simulink model "PassengerCar"  (R2019b)
settings: Solver=ode1  StartTime=0  StopTime=25  FixedStep=1.0000000000000000e-003  RelTol=1e-3
InitFcn:
  | sampleTime = str2double(get_param(bdroot, 'FixedStep'));
undefined symbols (not defined in the file or in its folder): AccPedalPos, BrakePedalPos, BrakeSwitch, DiscIntNeverNeededParam, DYNA4, EngSpd, IgnitionSwitch, InitialGear, InitialSpeed, IntendedEngTrq, LeftIndicator, MainBrakePress, MaxGear, MDL, MinGear, RefAcc, RefLane, RefLatPos, RefPath, RefPathCurv, RefSpd, RefSpdPreview, RefSpdRetrospect, RightIndicator, SteeringWheelAng, SteeringWheelTrq, UserDefinedRefValue, vm_const
libraries: UtilitiesLibrary x31, simulink x18, WheelSystemModules x13, LongitudinalControllerModules x13, LateralControllerModules x7, AnimationBusselectorModules x5, EnvironmentModules x5, BasicEngineControlModules x5, MiscellaneousControlModules x5, Animation3Modules x4, AuxiliariesModules x4, TireModules x4
(part 32 of 39)

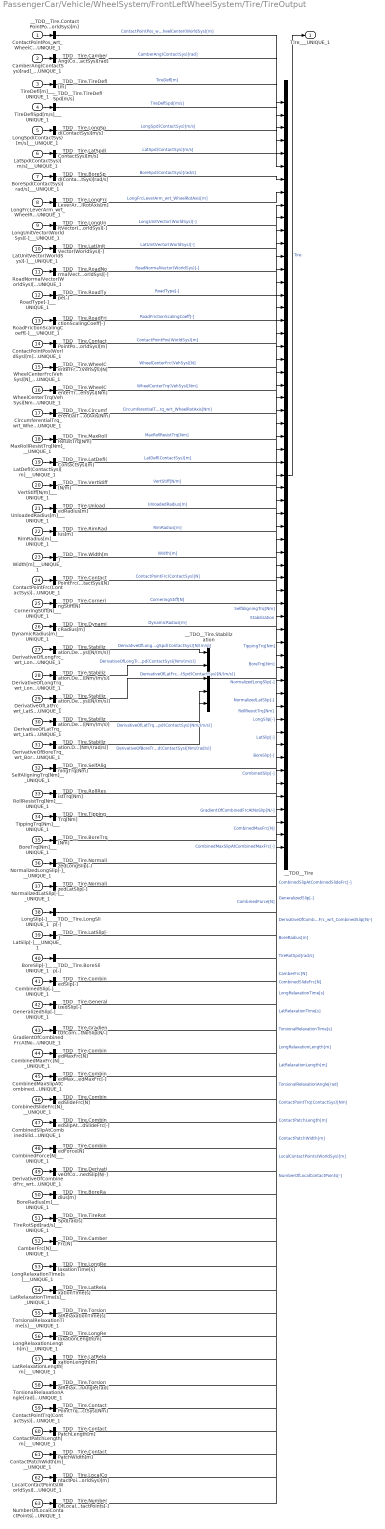
== system PassengerCar/Vehicle/WheelSystem/FrontLeftWheelSystem/Tire/TireOutput ==
  ContactPointPos_wrt_WheelCenter(WorldSys)[m]___UNIQUE_1 : Inport  Description=|  PortDimensions=[3]
      | <name>ContactPointPos_wrt_WheelCenter(WorldSys)[m]</name>
      | <comment></comment>
  CamberAng(ContactSys)[rad]___UNIQUE_1 : Inport  Description=|  Port=2  PortDimensions=[1]
      | <name>CamberAng(ContactSys)[rad]</name>
      | <comment></comment>
  TireDefl[m]___UNIQUE_1 : Inport  Description=|  Port=3  PortDimensions=[1]
      | <name>TireDefl[m]</name>
      | <comment></comment>
  TireDeflSpd[m/s]___UNIQUE_1 : Inport  Description=|  Port=4  PortDimensions=[1]
      | <name>TireDeflSpd[m/s]</name>
      | <comment></comment>
  LongSpd(ContactSys)[m/s]___UNIQUE_1 : Inport  Description=|  Port=5  PortDimensions=[1]
      | <name>LongSpd(ContactSys)[m/s]</name>
      | <comment></comment>
  LatSpd(ContactSys)[m/s]___UNIQUE_1 : Inport  Description=|  Port=6  PortDimensions=[1]
      | <name>LatSpd(ContactSys)[m/s]</name>
      | <comment></comment>
  BoreSpd(ContactSys)[rad/s]___UNIQUE_1 : Inport  Description=|  Port=7  PortDimensions=[1]
      | <name>BoreSpd(ContactSys)[rad/s]</name>
      | <comment></comment>
  LongFrcLeverArm_wrt_WheelRotAxis[m]___UNIQUE_1 : Inport  Description=|  Port=8  PortDimensions=[1]
      | <name>LongFrcLeverArm_wrt_WheelRotAxis[m]</name>
      | <comment></comment>
  LongUnitVector(WorldSys)[-]___UNIQUE_1 : Inport  Description=|  Port=9  PortDimensions=[3]
      | <name>LongUnitVector(WorldSys)[-]</name>
      | <comment></comment>
  LatUnitVector(WorldSys)[-]___UNIQUE_1 : Inport  Description=|  Port=10  PortDimensions=[3]
      | <name>LatUnitVector(WorldSys)[-]</name>
      | <comment></comment>
  RoadNormalVector(WorldSys)[-]___UNIQUE_1 : Inport  Description=|  Port=11  PortDimensions=[3]
      | <name>RoadNormalVector(WorldSys)[-]</name>
      | <comment></comment>
  RoadType[-]___UNIQUE_1 : Inport  Description=|  Port=12  PortDimensions=[1]
      | <name>RoadType[-]</name>
      | <comment></comment>
  RoadFrictionScalingCoeff[-]___UNIQUE_1 : Inport  Description=|  Port=13  PortDimensions=[1]
      | <name>RoadFrictionScalingCoeff[-]</name>
      | <comment></comment>
  ContactPointPos(WorldSys)[m]___UNIQUE_1 : Inport  Description=|  Port=14  PortDimensions=[3]
      | <name>ContactPointPos(WorldSys)[m]</name>
      | <comment></comment>
  WheelCenterFrc(VehSys)[N]___UNIQUE_1 : Inport  Description=|  Port=15  PortDimensions=[3]
      | <name>WheelCenterFrc(VehSys)[N]</name>
      | <comment></comment>
  WheelCenterTrq(VehSys)[Nm]___UNIQUE_1 : Inport  Description=|  Port=16  PortDimensions=[3]
      | <name>WheelCenterTrq(VehSys)[Nm]</name>
      | <comment></comment>
  CircumferentialTrq_wrt_WheelRotAxis[Nm]___UNIQUE_1 : Inport  Description=|  Port=17  PortDimensions=[1]
      | <name>CircumferentialTrq_wrt_WheelRotAxis[Nm]</name>
      | <comment></comment>
  MaxRollResistTrq[Nm]___UNIQUE_1 : Inport  Description=|  Port=18  PortDimensions=[1]
      | <name>MaxRollResistTrq[Nm]</name>
      | <comment></comment>
  LatDefl(ContactSys)[m]___UNIQUE_1 : Inport  Description=|  Port=19  PortDimensions=[1]
      | <name>LatDefl(ContactSys)[m]</name>
      | <comment></comment>
  VertStiff[N/m]___UNIQUE_1 : Inport  Description=|  Port=20  PortDimensions=[1]
      | <name>VertStiff[N/m]</name>
      | <comment></comment>
  UnloadedRadius[m]___UNIQUE_1 : Inport  Description=|  Port=21  PortDimensions=[1]
      | <name>UnloadedRadius[m]</name>
      | <comment></comment>
  RimRadius[m]___UNIQUE_1 : Inport  Description=|  Port=22  PortDimensions=[1]
      | <name>RimRadius[m]</name>
      | <comment></comment>
  Width[m]___UNIQUE_1 : Inport  Description=|  Port=23  PortDimensions=[1]
      | <name>Width[m]</name>
      | <comment></comment>
  ContactPointFrc(ContactSys)[N]___UNIQUE_1 : Inport  Description=|  Port=24  PortDimensions=[3]
      | <name>ContactPointFrc(ContactSys)[N]</name>
      | <comment></comment>
  CorneringStiff[N]___UNIQUE_1 : Inport  Description=|  Port=25  PortDimensions=[1]
      | <name>CorneringStiff[N]</name>
      | <comment></comment>
  DynamicRadius[m]___UNIQUE_1 : Inport  Description=|  Port=26  PortDimensions=[1]
      | <name>DynamicRadius[m]</name>
      | <comment></comment>
  DerivativeOfLongFrc_wrt_LongSpd(ContactSys)[N/(m/s)]___UNIQUE_1 : Inport  Description=|  Port=27  PortDimensions=[1]
      | <name>Stabilization.DerivativeOfLongFrc_wrt_LongSpd(ContactSys)[N/(m/s)]</name>
      | <comment></comment>
  DerivativeOfLongTrq_wrt_LongSpd(ContactSys)[Nm/(m/s)]___UNIQUE_1 : Inport  Description=|  Port=28  PortDimensions=[1]
      | <name>Stabilization.DerivativeOfLongTrq_wrt_LongSpd(ContactSys)[Nm/(m/s)]</name>
      | <comment></comment>
  DerivativeOfLatFrc_wrt_LatSpd(ContactSys)[N/(m/s)]___UNIQUE_1 : Inport  Description=|  Port=29  PortDimensions=[1]
      | <name>Stabilization.DerivativeOfLatFrc_wrt_LatSpd(ContactSys)[N/(m/s)]</name>
      | <comment></comment>
  DerivativeOfLatTrq_wrt_LatSpd(ContactSys)[Nm/(m/s)]___UNIQUE_1 : Inport  Description=|  Port=30  PortDimensions=[1]
      | <name>Stabilization.DerivativeOfLatTrq_wrt_LatSpd(ContactSys)[Nm/(m/s)]</name>
      | <comment></comment>
  DerivativeOfBoreTrq_wrt_BoreSpd(ContactSys)[Nm/(rad/s)]___UNIQUE_1 : Inport  Description=|  Port=31  PortDimensions=[1]
      | <name>Stabilization.DerivativeOfBoreTrq_wrt_BoreSpd(ContactSys)[Nm/(rad/s)]</name>
      | <comment></comment>
  SelfAligningTrq[Nm]___UNIQUE_1 : Inport  Description=|  Port=32  PortDimensions=[1]
      | <name>SelfAligningTrq[Nm]</name>
      | <comment></comment>
  RollResistTrq[Nm]___UNIQUE_1 : Inport  Description=|  Port=33  PortDimensions=[1]
      | <name>RollResistTrq[Nm]</name>
      | <comment></comment>
  TippingTrq[Nm]___UNIQUE_1 : Inport  Description=|  Port=34  PortDimensions=[1]
      | <name>TippingTrq[Nm]</name>
      | <comment></comment>
  BoreTrq[Nm]___UNIQUE_1 : Inport  Description=|  Port=35  PortDimensions=[1]
      | <name>BoreTrq[Nm]</name>
      | <comment></comment>
  NormalizedLongSlip[-]___UNIQUE_1 : Inport  Description=|  Port=36  PortDimensions=[1]
      | <name>NormalizedLongSlip[-]</name>
      | <comment></comment>
  NormalizedLatSlip[-]___UNIQUE_1 : Inport  Description=|  Port=37  PortDimensions=[1]
      | <name>NormalizedLatSlip[-]</name>
      | <comment></comment>
  LongSlip[-]___UNIQUE_1 : Inport  Description=|  Port=38  PortDimensions=[1]
      | <name>LongSlip[-]</name>
      | <comment></comment>
  LatSlip[-]___UNIQUE_1 : Inport  Description=|  Port=39  PortDimensions=[1]
      | <name>LatSlip[-]</name>
      | <comment></comment>
  BoreSlip[-]___UNIQUE_1 : Inport  Description=|  Port=40  PortDimensions=[1]
      | <name>BoreSlip[-]</name>
      | <comment></comment>
  CombinedSlip[-]___UNIQUE_1 : Inport  Description=|  Port=41  PortDimensions=[1]
      | <name>CombinedSlip[-]</name>
      | <comment></comment>
  GeneralizedSlip[-]___UNIQUE_1 : Inport  Description=|  Port=42  PortDimensions=[1]
      | <name>GeneralizedSlip[-]</name>
      | <comment></comment>
  GradientOfCombinedFrcAtNoSlip[N/-]___UNIQUE_1 : Inport  Description=|  Port=43  PortDimensions=[1]
      | <name>GradientOfCombinedFrcAtNoSlip[N/-]</name>
      | <comment></comment>
  CombinedMaxFrc[N]___UNIQUE_1 : Inport  Description=|  Port=44  PortDimensions=[1]
      | <name>CombinedMaxFrc[N]</name>
      | <comment></comment>
  CombinedMaxSlipAtCombinedMaxFrc[-]___UNIQUE_1 : Inport  Description=|  Port=45  PortDimensions=[1]
      | <name>CombinedMaxSlipAtCombinedMaxFrc[-]</name>
      | <comment></comment>
  CombinedSlideFrc[N]___UNIQUE_1 : Inport  Description=|  Port=46  PortDimensions=[1]
      | <name>CombinedSlideFrc[N]</name>
      | <comment></comment>
  CombinedSlipAtCombinedSlideFrc[-]___UNIQUE_1 : Inport  Description=|  Port=47  PortDimensions=[1]
      | <name>CombinedSlipAtCombinedSlideFrc[-]</name>
      | <comment></comment>
  CombinedForce[N]___UNIQUE_1 : Inport  Description=|  Port=48  PortDimensions=[1]
      | <name>CombinedForce[N]</name>
      | <comment></comment>
  DerivativeOfCombinedFrc_wrt_CombinedSlip[N/-]___UNIQUE_1 : Inport  Description=|  Port=49  PortDimensions=[1]
      | <name>DerivativeOfCombinedFrc_wrt_CombinedSlip[N/-]</name>
      | <comment></comment>
  BoreRadius[m]___UNIQUE_1 : Inport  Description=|  Port=50  PortDimensions=[1]
      | <name>BoreRadius[m]</name>
      | <comment></comment>
  TireRotSpd[rad/s]___UNIQUE_1 : Inport  Description=|  Port=51  PortDimensions=[1]
      | <name>TireRotSpd[rad/s]</name>
      | <comment></comment>
  CamberFrc[N]___UNIQUE_1 : Inport  Description=|  Port=52  PortDimensions=[1]
      | <name>CamberFrc[N]</name>
      | <comment></comment>
  LongRelaxationTime[s]___UNIQUE_1 : Inport  Description=|  Port=53  PortDimensions=[1]
      | <name>LongRelaxationTime[s]</name>
      | <comment></comment>
  LatRelaxationTime[s]___UNIQUE_1 : Inport  Description=|  Port=54  PortDimensions=[1]
      | <name>LatRelaxationTime[s]</name>
      | <comment></comment>
  TorsionalRelaxationTime[s]___UNIQUE_1 : Inport  Description=|  Port=55  PortDimensions=[1]
      | <name>TorsionalRelaxationTime[s]</name>
      | <comment></comment>
  LongRelaxationLength[m]___UNIQUE_1 : Inport  Description=|  Port=56  PortDimensions=[1]
      | <name>LongRelaxationLength[m]</name>
      | <comment></comment>
  LatRelaxationLength[m]___UNIQUE_1 : Inport  Description=|  Port=57  PortDimensions=[1]
      | <name>LatRelaxationLength[m]</name>
      | <comment></comment>
  TorsionalRelaxationAngle[rad]___UNIQUE_1 : Inport  Description=|  Port=58  PortDimensions=[1]
      | <name>TorsionalRelaxationAngle[rad]</name>
      | <comment></comment>
  ContactPointTrq(ContactSys)[Nm]___UNIQUE_1 : Inport  Description=|  Port=59  PortDimensions=[3]
      | <name>ContactPointTrq(ContactSys)[Nm]</name>
      | <comment></comment>
  ContactPatchLength[m]___UNIQUE_1 : Inport  Description=|  Port=60  PortDimensions=[1]
      | <name>ContactPatchLength[m]</name>
      | <comment></comment>
  ContactPatchWidth[m]___UNIQUE_1 : Inport  Description=|  Port=61  PortDimensions=[1]
      | <name>ContactPatchWidth[m]</name>
      | <comment></comment>
  LocalContactPoints(WorldSys)[m]___UNIQUE_1 : Inport  Description=|  Port=62  PortDimensions=[12]
      | <name>LocalContactPoints(WorldSys)[m]</name>
      | <comment></comment>
  NumberOfLocalContactPoints[-]___UNIQUE_1 : Inport  Description=|  Port=63  PortDimensions=[1]
      | <name>NumberOfLocalContactPoints[-]</name>
      | <comment></comment>
  __TDD__Tire.BoreRadius[m] : Demux  Outputs=[1]
  __TDD__Tire.BoreSlip[-] : Demux  Outputs=[1]
  __TDD__Tire.BoreSpd(ContactSys)[rad/s] : Demux  Outputs=[1]
  __TDD__Tire.BoreTrq[Nm] : Demux  Outputs=[1]
  __TDD__Tire.CamberAng(ContactSys)[rad] : Demux  Outputs=[1]
  __TDD__Tire.CamberFrc[N] : Demux  Outputs=[1]
  __TDD__Tire.CircumferentialTrq_wrt_WheelRotAxis[Nm] : Demux  Outputs=[1]
  __TDD__Tire.CombinedForce[N] : Demux  Outputs=[1]
  __TDD__Tire.CombinedMaxFrc[N] : Demux  Outputs=[1]
  __TDD__Tire.CombinedMaxSlipAtCombinedMaxFrc[-] : Demux  Outputs=[1]
  __TDD__Tire.CombinedSlideFrc[N] : Demux  Outputs=[1]
  __TDD__Tire.CombinedSlipAtCombinedSlideFrc[-] : Demux  Outputs=[1]
  __TDD__Tire.CombinedSlip[-] : Demux  Outputs=[1]
  __TDD__Tire.ContactPatchLength[m] : Demux  Outputs=[1]
  __TDD__Tire.ContactPatchWidth[m] : Demux  Outputs=[1]
  __TDD__Tire.ContactPointFrc(ContactSys)[N] : Demux  Outputs=[3]
  __TDD__Tire.ContactPointPos(WorldSys)[m] : Demux  Outputs=[3]
  __TDD__Tire.ContactPointPos_wrt_WheelCenter(WorldSys)[m] : Demux  Outputs=[3]
  __TDD__Tire.ContactPointTrq(ContactSys)[Nm] : Demux  Outputs=[3]
  __TDD__Tire.CorneringStiff[N] : Demux  Outputs=[1]
  __TDD__Tire.DerivativeOfCombinedFrc_wrt_CombinedSlip[N/-] : Demux  Outputs=[1]
  __TDD__Tire.DynamicRadius[m] : Demux  Outputs=[1]
  __TDD__Tire.GeneralizedSlip[-] : Demux  Outputs=[1]
  __TDD__Tire.GradientOfCombinedFrcAtNoSlip[N/-] : Demux  Outputs=[1]
  __TDD__Tire.LatDefl(ContactSys)[m] : Demux  Outputs=[1]
  __TDD__Tire.LatRelaxationLength[m] : Demux  Outputs=[1]
  __TDD__Tire.LatRelaxationTime[s] : Demux  Outputs=[1]
  __TDD__Tire.LatSlip[-] : Demux  Outputs=[1]
  __TDD__Tire.LatSpd(ContactSys)[m/s] : Demux  Outputs=[1]
  __TDD__Tire.LatUnitVector(WorldSys)[-] : Demux  Outputs=[3]
  __TDD__Tire.LocalContactPoints(WorldSys)[m] : Demux  Outputs=[12]
  __TDD__Tire.LongFrcLeverArm_wrt_WheelRotAxis[m] : Demux  Outputs=[1]
  __TDD__Tire.LongRelaxationLength[m] : Demux  Outputs=[1]
  __TDD__Tire.LongRelaxationTime[s] : Demux  Outputs=[1]
  __TDD__Tire.LongSlip[-] : Demux  Outputs=[1]
  __TDD__Tire.LongSpd(ContactSys)[m/s] : Demux  Outputs=[1]
  __TDD__Tire.LongUnitVector(WorldSys)[-] : Demux  Outputs=[3]
  __TDD__Tire.MaxRollResistTrq[Nm] : Demux  Outputs=[1]
  __TDD__Tire.NormalizedLatSlip[-] : Demux  Outputs=[1]
  __TDD__Tire.NormalizedLongSlip[-] : Demux  Outputs=[1]
  __TDD__Tire.NumberOfLocalContactPoints[-] : Demux  Outputs=[1]
  __TDD__Tire.RimRadius[m] : Demux  Outputs=[1]
  __TDD__Tire.RoadFrictionScalingCoeff[-] : Demux  Outputs=[1]
  __TDD__Tire.RoadNormalVector(WorldSys)[-] : Demux  Outputs=[3]
  __TDD__Tire.RoadType[-] : Demux  Outputs=[1]
  __TDD__Tire.RollResistTrq[Nm] : Demux  Outputs=[1]
  __TDD__Tire.SelfAligningTrq[Nm] : Demux  Outputs=[1]
  __TDD__Tire.Stabilization.DerivativeOfBoreTrq_wrt_BoreSpd(ContactSys)[Nm/(rad/s)] : Demux  Outputs=[1]
  __TDD__Tire.Stabilization.DerivativeOfLatFrc_wrt_LatSpd(ContactSys)[N/(m/s)] : Demux  Outputs=[1]
  __TDD__Tire.Stabilization.DerivativeOfLatTrq_wrt_LatSpd(ContactSys)[Nm/(m/s)] : Demux  Outputs=[1]
  __TDD__Tire.Stabilization.DerivativeOfLongFrc_wrt_LongSpd(ContactSys)[N/(m/s)] : Demux  Outputs=[1]
  __TDD__Tire.Stabilization.DerivativeOfLongTrq_wrt_LongSpd(ContactSys)[Nm/(m/s)] : Demux  Outputs=[1]
  __TDD__Tire.TippingTrq[Nm] : Demux  Outputs=[1]
  __TDD__Tire.TireDeflSpd[m/s] : Demux  Outputs=[1]
  __TDD__Tire.TireDefl[m] : Demux  Outputs=[1]
  __TDD__Tire.TireRotSpd[rad/s] : Demux  Outputs=[1]
  __TDD__Tire.TorsionalRelaxationAngle[rad] : Demux  Outputs=[1]
  __TDD__Tire.TorsionalRelaxationTime[s] : Demux  Outputs=[1]
  __TDD__Tire.UnloadedRadius[m] : Demux  Outputs=[1]
  __TDD__Tire.VertStiff[N/m] : Demux  Outputs=[1]
  __TDD__Tire.WheelCenterFrc(VehSys)[N] : Demux  Outputs=[3]
  __TDD__Tire.WheelCenterTrq(VehSys)[Nm] : Demux  Outputs=[3]
  __TDD__Tire.Width[m] : Demux  Outputs=[1]
  __TDO__Tire : BusCreator  Inputs=59
  __TDO__Tire.Stabilization : BusCreator  Inputs=5
  Tire___UNIQUE_1 : Outport  Description=|  PortDimensions=[92]  VectorParamsAs1DForOutWhenUnconnected=off
      | <name>ContactPointPos_wrt_WheelCenter(WorldSys)[m]</name>
      | <comment></comment>
  wires:
  ContactPointPos_wrt_WheelCenter(WorldSys)[m]___UNIQUE_1/1 -> __TDD__Tire.ContactPointPos_wrt_WheelCenter(WorldSys)[m]/1
  __TDD__Tire.ContactPointPos_wrt_WheelCenter(WorldSys)[m]/1 -> __TDO__Tire/1  "ContactPointPos_wrt_WheelCenter(WorldSys)[m]"
  CamberAng(ContactSys)[rad]___UNIQUE_1/1 -> __TDD__Tire.CamberAng(ContactSys)[rad]/1
  __TDD__Tire.CamberAng(ContactSys)[rad]/1 -> __TDO__Tire/2  "CamberAng(ContactSys)[rad]"
  TireDefl[m]___UNIQUE_1/1 -> __TDD__Tire.TireDefl[m]/1
  __TDD__Tire.TireDefl[m]/1 -> __TDO__Tire/3  "TireDefl[m]"
  TireDeflSpd[m/s]___UNIQUE_1/1 -> __TDD__Tire.TireDeflSpd[m/s]/1
  __TDD__Tire.TireDeflSpd[m/s]/1 -> __TDO__Tire/4  "TireDeflSpd[m/s]"
  LongSpd(ContactSys)[m/s]___UNIQUE_1/1 -> __TDD__Tire.LongSpd(ContactSys)[m/s]/1
  __TDD__Tire.LongSpd(ContactSys)[m/s]/1 -> __TDO__Tire/5  "LongSpd(ContactSys)[m/s]"
  LatSpd(ContactSys)[m/s]___UNIQUE_1/1 -> __TDD__Tire.LatSpd(ContactSys)[m/s]/1
  __TDD__Tire.LatSpd(ContactSys)[m/s]/1 -> __TDO__Tire/6  "LatSpd(ContactSys)[m/s]"
  BoreSpd(ContactSys)[rad/s]___UNIQUE_1/1 -> __TDD__Tire.BoreSpd(ContactSys)[rad/s]/1
  __TDD__Tire.BoreSpd(ContactSys)[rad/s]/1 -> __TDO__Tire/7  "BoreSpd(ContactSys)[rad/s]"
  LongFrcLeverArm_wrt_WheelRotAxis[m]___UNIQUE_1/1 -> __TDD__Tire.LongFrcLeverArm_wrt_WheelRotAxis[m]/1
  __TDD__Tire.LongFrcLeverArm_wrt_WheelRotAxis[m]/1 -> __TDO__Tire/8  "LongFrcLeverArm_wrt_WheelRotAxis[m]"
  LongUnitVector(WorldSys)[-]___UNIQUE_1/1 -> __TDD__Tire.LongUnitVector(WorldSys)[-]/1
  __TDD__Tire.LongUnitVector(WorldSys)[-]/1 -> __TDO__Tire/9  "LongUnitVector(WorldSys)[-]"
  LatUnitVector(WorldSys)[-]___UNIQUE_1/1 -> __TDD__Tire.LatUnitVector(WorldSys)[-]/1
  __TDD__Tire.LatUnitVector(WorldSys)[-]/1 -> __TDO__Tire/10  "LatUnitVector(WorldSys)[-]"
  RoadNormalVector(WorldSys)[-]___UNIQUE_1/1 -> __TDD__Tire.RoadNormalVector(WorldSys)[-]/1
  __TDD__Tire.RoadNormalVector(WorldSys)[-]/1 -> __TDO__Tire/11  "RoadNormalVector(WorldSys)[-]"
  RoadType[-]___UNIQUE_1/1 -> __TDD__Tire.RoadType[-]/1
  __TDD__Tire.RoadType[-]/1 -> __TDO__Tire/12  "RoadType[-]"
  RoadFrictionScalingCoeff[-]___UNIQUE_1/1 -> __TDD__Tire.RoadFrictionScalingCoeff[-]/1
  __TDD__Tire.RoadFrictionScalingCoeff[-]/1 -> __TDO__Tire/13  "RoadFrictionScalingCoeff[-]"
  ContactPointPos(WorldSys)[m]___UNIQUE_1/1 -> __TDD__Tire.ContactPointPos(WorldSys)[m]/1
  __TDD__Tire.ContactPointPos(WorldSys)[m]/1 -> __TDO__Tire/14  "ContactPointPos(WorldSys)[m]"
  WheelCenterFrc(VehSys)[N]___UNIQUE_1/1 -> __TDD__Tire.WheelCenterFrc(VehSys)[N]/1
  __TDD__Tire.WheelCenterFrc(VehSys)[N]/1 -> __TDO__Tire/15  "WheelCenterFrc(VehSys)[N]"
  WheelCenterTrq(VehSys)[Nm]___UNIQUE_1/1 -> __TDD__Tire.WheelCenterTrq(VehSys)[Nm]/1
  __TDD__Tire.WheelCenterTrq(VehSys)[Nm]/1 -> __TDO__Tire/16  "WheelCenterTrq(VehSys)[Nm]"
  CircumferentialTrq_wrt_WheelRotAxis[Nm]___UNIQUE_1/1 -> __TDD__Tire.CircumferentialTrq_wrt_WheelRotAxis[Nm]/1
  __TDD__Tire.CircumferentialTrq_wrt_WheelRotAxis[Nm]/1 -> __TDO__Tire/17  "CircumferentialTrq_wrt_WheelRotAxis[Nm]"
  MaxRollResistTrq[Nm]___UNIQUE_1/1 -> __TDD__Tire.MaxRollResistTrq[Nm]/1
  __TDD__Tire.MaxRollResistTrq[Nm]/1 -> __TDO__Tire/18  "MaxRollResistTrq[Nm]"
  LatDefl(ContactSys)[m]___UNIQUE_1/1 -> __TDD__Tire.LatDefl(ContactSys)[m]/1
  __TDD__Tire.LatDefl(ContactSys)[m]/1 -> __TDO__Tire/19  "LatDefl(ContactSys)[m]"
  VertStiff[N/m]___UNIQUE_1/1 -> __TDD__Tire.VertStiff[N/m]/1
  __TDD__Tire.VertStiff[N/m]/1 -> __TDO__Tire/20  "VertStiff[N/m]"
  UnloadedRadius[m]___UNIQUE_1/1 -> __TDD__Tire.UnloadedRadius[m]/1
  __TDD__Tire.UnloadedRadius[m]/1 -> __TDO__Tire/21  "UnloadedRadius[m]"
  RimRadius[m]___UNIQUE_1/1 -> __TDD__Tire.RimRadius[m]/1
  __TDD__Tire.RimRadius[m]/1 -> __TDO__Tire/22  "RimRadius[m]"
  Width[m]___UNIQUE_1/1 -> __TDD__Tire.Width[m]/1
  __TDD__Tire.Width[m]/1 -> __TDO__Tire/23  "Width[m]"
  ContactPointFrc(ContactSys)[N]___UNIQUE_1/1 -> __TDD__Tire.ContactPointFrc(ContactSys)[N]/1
  __TDD__Tire.ContactPointFrc(ContactSys)[N]/1 -> __TDO__Tire/24  "ContactPointFrc(ContactSys)[N]"
  CorneringStiff[N]___UNIQUE_1/1 -> __TDD__Tire.CorneringStiff[N]/1
  __TDD__Tire.CorneringStiff[N]/1 -> __TDO__Tire/25  "CorneringStiff[N]"
  DynamicRadius[m]___UNIQUE_1/1 -> __TDD__Tire.DynamicRadius[m]/1
  __TDD__Tire.DynamicRadius[m]/1 -> __TDO__Tire/26  "DynamicRadius[m]"
  DerivativeOfLongFrc_wrt_LongSpd(ContactSys)[N/(m/s)]___UNIQUE_1/1 -> __TDD__Tire.Stabilization.DerivativeOfLongFrc_wrt_LongSpd(ContactSys)[N/(m/s)]/1
  __TDD__Tire.Stabilization.DerivativeOfLongFrc_wrt_LongSpd(ContactSys)[N/(m/s)]/1 -> __TDO__Tire.Stabilization/1  "DerivativeOfLongFrc_wrt_LongSpd(ContactSys)[N/(m/s)]"
  __TDO__Tire.Stabilization/1 -> __TDO__Tire/27  "Stabilization"
  DerivativeOfLongTrq_wrt_LongSpd(ContactSys)[Nm/(m/s)]___UNIQUE_1/1 -> __TDD__Tire.Stabilization.DerivativeOfLongTrq_wrt_LongSpd(ContactSys)[Nm/(m/s)]/1
  __TDD__Tire.Stabilization.DerivativeOfLongTrq_wrt_LongSpd(ContactSys)[Nm/(m/s)]/1 -> __TDO__Tire.Stabilization/2  "DerivativeOfLongTrq_wrt_LongSpd(ContactSys)[Nm/(m/s)]"
  DerivativeOfLatFrc_wrt_LatSpd(ContactSys)[N/(m/s)]___UNIQUE_1/1 -> __TDD__Tire.Stabilization.DerivativeOfLatFrc_wrt_LatSpd(ContactSys)[N/(m/s)]/1
  __TDD__Tire.Stabilization.DerivativeOfLatFrc_wrt_LatSpd(ContactSys)[N/(m/s)]/1 -> __TDO__Tire.Stabilization/3  "DerivativeOfLatFrc_wrt_LatSpd(ContactSys)[N/(m/s)]"
  DerivativeOfLatTrq_wrt_LatSpd(ContactSys)[Nm/(m/s)]___UNIQUE_1/1 -> __TDD__Tire.Stabilization.DerivativeOfLatTrq_wrt_LatSpd(ContactSys)[Nm/(m/s)]/1
  __TDD__Tire.Stabilization.DerivativeOfLatTrq_wrt_LatSpd(ContactSys)[Nm/(m/s)]/1 -> __TDO__Tire.Stabilization/4  "DerivativeOfLatTrq_wrt_LatSpd(ContactSys)[Nm/(m/s)]"
  DerivativeOfBoreTrq_wrt_BoreSpd(ContactSys)[Nm/(rad/s)]___UNIQUE_1/1 -> __TDD__Tire.Stabilization.DerivativeOfBoreTrq_wrt_BoreSpd(ContactSys)[Nm/(rad/s)]/1
  __TDD__Tire.Stabilization.DerivativeOfBoreTrq_wrt_BoreSpd(ContactSys)[Nm/(rad/s)]/1 -> __TDO__Tire.Stabilization/5  "DerivativeOfBoreTrq_wrt_BoreSpd(ContactSys)[Nm/(rad/s)]"
  SelfAligningTrq[Nm]___UNIQUE_1/1 -> __TDD__Tire.SelfAligningTrq[Nm]/1
  __TDD__Tire.SelfAligningTrq[Nm]/1 -> __TDO__Tire/28  "SelfAligningTrq[Nm]"
  RollResistTrq[Nm]___UNIQUE_1/1 -> __TDD__Tire.RollResistTrq[Nm]/1
  __TDD__Tire.RollResistTrq[Nm]/1 -> __TDO__Tire/29  "RollResistTrq[Nm]"
  TippingTrq[Nm]___UNIQUE_1/1 -> __TDD__Tire.TippingTrq[Nm]/1
  __TDD__Tire.TippingTrq[Nm]/1 -> __TDO__Tire/30  "TippingTrq[Nm]"
  BoreTrq[Nm]___UNIQUE_1/1 -> __TDD__Tire.BoreTrq[Nm]/1
  __TDD__Tire.BoreTrq[Nm]/1 -> __TDO__Tire/31  "BoreTrq[Nm]"
  NormalizedLongSlip[-]___UNIQUE_1/1 -> __TDD__Tire.NormalizedLongSlip[-]/1
  __TDD__Tire.NormalizedLongSlip[-]/1 -> __TDO__Tire/32  "NormalizedLongSlip[-]"
  NormalizedLatSlip[-]___UNIQUE_1/1 -> __TDD__Tire.NormalizedLatSlip[-]/1
  __TDD__Tire.NormalizedLatSlip[-]/1 -> __TDO__Tire/33  "NormalizedLatSlip[-]"
  LongSlip[-]___UNIQUE_1/1 -> __TDD__Tire.LongSlip[-]/1
  __TDD__Tire.LongSlip[-]/1 -> __TDO__Tire/34  "LongSlip[-]"
  LatSlip[-]___UNIQUE_1/1 -> __TDD__Tire.LatSlip[-]/1
  __TDD__Tire.LatSlip[-]/1 -> __TDO__Tire/35  "LatSlip[-]"
  BoreSlip[-]___UNIQUE_1/1 -> __TDD__Tire.BoreSlip[-]/1
  __TDD__Tire.BoreSlip[-]/1 -> __TDO__Tire/36  "BoreSlip[-]"
  CombinedSlip[-]___UNIQUE_1/1 -> __TDD__Tire.CombinedSlip[-]/1
  __TDD__Tire.CombinedSlip[-]/1 -> __TDO__Tire/37  "CombinedSlip[-]"
  GeneralizedSlip[-]___UNIQUE_1/1 -> __TDD__Tire.GeneralizedSlip[-]/1
  __TDD__Tire.GeneralizedSlip[-]/1 -> __TDO__Tire/38  "GeneralizedSlip[-]"
  GradientOfCombinedFrcAtNoSlip[N/-]___UNIQUE_1/1 -> __TDD__Tire.GradientOfCombinedFrcAtNoSlip[N/-]/1
  __TDD__Tire.GradientOfCombinedFrcAtNoSlip[N/-]/1 -> __TDO__Tire/39  "GradientOfCombinedFrcAtNoSlip[N/-]"
  CombinedMaxFrc[N]___UNIQUE_1/1 -> __TDD__Tire.CombinedMaxFrc[N]/1
  __TDD__Tire.CombinedMaxFrc[N]/1 -> __TDO__Tire/40  "CombinedMaxFrc[N]"
  CombinedMaxSlipAtCombinedMaxFrc[-]___UNIQUE_1/1 -> __TDD__Tire.CombinedMaxSlipAtCombinedMaxFrc[-]/1
  __TDD__Tire.CombinedMaxSlipAtCombinedMaxFrc[-]/1 -> __TDO__Tire/41  "CombinedMaxSlipAtCombinedMaxFrc[-]"
  CombinedSlideFrc[N]___UNIQUE_1/1 -> __TDD__Tire.CombinedSlideFrc[N]/1
  __TDD__Tire.CombinedSlideFrc[N]/1 -> __TDO__Tire/42  "CombinedSlideFrc[N]"
  CombinedSlipAtCombinedSlideFrc[-]___UNIQUE_1/1 -> __TDD__Tire.CombinedSlipAtCombinedSlideFrc[-]/1
  __TDD__Tire.CombinedSlipAtCombinedSlideFrc[-]/1 -> __TDO__Tire/43  "CombinedSlipAtCombinedSlideFrc[-]"
  CombinedForce[N]___UNIQUE_1/1 -> __TDD__Tire.CombinedForce[N]/1
  __TDD__Tire.CombinedForce[N]/1 -> __TDO__Tire/44  "CombinedForce[N]"
  DerivativeOfCombinedFrc_wrt_CombinedSlip[N/-]___UNIQUE_1/1 -> __TDD__Tire.DerivativeOfCombinedFrc_wrt_CombinedSlip[N/-]/1
  __TDD__Tire.DerivativeOfCombinedFrc_wrt_CombinedSlip[N/-]/1 -> __TDO__Tire/45  "DerivativeOfCombinedFrc_wrt_CombinedSlip[N/-]"
  BoreRadius[m]___UNIQUE_1/1 -> __TDD__Tire.BoreRadius[m]/1
  __TDD__Tire.BoreRadius[m]/1 -> __TDO__Tire/46  "BoreRadius[m]"
  TireRotSpd[rad/s]___UNIQUE_1/1 -> __TDD__Tire.TireRotSpd[rad/s]/1
  __TDD__Tire.TireRotSpd[rad/s]/1 -> __TDO__Tire/47  "TireRotSpd[rad/s]"
  CamberFrc[N]___UNIQUE_1/1 -> __TDD__Tire.CamberFrc[N]/1
  __TDD__Tire.CamberFrc[N]/1 -> __TDO__Tire/48  "CamberFrc[N]"
  LongRelaxationTime[s]___UNIQUE_1/1 -> __TDD__Tire.LongRelaxationTime[s]/1
  __TDD__Tire.LongRelaxationTime[s]/1 -> __TDO__Tire/49  "LongRelaxationTime[s]"
  LatRelaxationTime[s]___UNIQUE_1/1 -> __TDD__Tire.LatRelaxationTime[s]/1
  __TDD__Tire.LatRelaxationTime[s]/1 -> __TDO__Tire/50  "LatRelaxationTime[s]"
  TorsionalRelaxationTime[s]___UNIQUE_1/1 -> __TDD__Tire.TorsionalRelaxationTime[s]/1
  __TDD__Tire.TorsionalRelaxationTime[s]/1 -> __TDO__Tire/51  "TorsionalRelaxationTime[s]"
  LongRelaxationLength[m]___UNIQUE_1/1 -> __TDD__Tire.LongRelaxationLength[m]/1
  __TDD__Tire.LongRelaxationLength[m]/1 -> __TDO__Tire/52  "LongRelaxationLength[m]"
  LatRelaxationLength[m]___UNIQUE_1/1 -> __TDD__Tire.LatRelaxationLength[m]/1
  __TDD__Tire.LatRelaxationLength[m]/1 -> __TDO__Tire/53  "LatRelaxationLength[m]"
  TorsionalRelaxationAngle[rad]___UNIQUE_1/1 -> __TDD__Tire.TorsionalRelaxationAngle[rad]/1
  __TDD__Tire.TorsionalRelaxationAngle[rad]/1 -> __TDO__Tire/54  "TorsionalRelaxationAngle[rad]"
  ContactPointTrq(ContactSys)[Nm]___UNIQUE_1/1 -> __TDD__Tire.ContactPointTrq(ContactSys)[Nm]/1
  __TDD__Tire.ContactPointTrq(ContactSys)[Nm]/1 -> __TDO__Tire/55  "ContactPointTrq(ContactSys)[Nm]"
  ContactPatchLength[m]___UNIQUE_1/1 -> __TDD__Tire.ContactPatchLength[m]/1
  __TDD__Tire.ContactPatchLength[m]/1 -> __TDO__Tire/56  "ContactPatchLength[m]"
  ContactPatchWidth[m]___UNIQUE_1/1 -> __TDD__Tire.ContactPatchWidth[m]/1
  __TDD__Tire.ContactPatchWidth[m]/1 -> __TDO__Tire/57  "ContactPatchWidth[m]"
  LocalContactPoints(WorldSys)[m]___UNIQUE_1/1 -> __TDD__Tire.LocalContactPoints(WorldSys)[m]/1
  __TDD__Tire.LocalContactPoints(WorldSys)[m]/1 -> __TDO__Tire/58  "LocalContactPoints(WorldSys)[m]"
  NumberOfLocalContactPoints[-]___UNIQUE_1/1 -> __TDD__Tire.NumberOfLocalContactPoints[-]/1
  __TDD__Tire.NumberOfLocalContactPoints[-]/1 -> __TDO__Tire/59  "NumberOfLocalContactPoints[-]"
  __TDO__Tire/1 -> Tire___UNIQUE_1/1  "Tire"

== system PassengerCar/Vehicle/WheelSystem/FrontRightWheelSystem/Tire/DynaComponentInfo ==

== system PassengerCar/Vehicle/WheelSystem/FrontRightWheelSystem/Tire/InputFromCTRL ==
  fromCTRL : Inport
  TDBusSelector : BusSelector  OutputSignals=AddRoadElev[m],RoadFrictionScaling[0_2],AddLongRoadSlope[-],AddLatRoadSlope[-],LocalRoadSysSwitch[0;1],RelInflPress[Pa]
  __TDD__AddLatRoadSlope[-] : Demux  Outputs=[1]
  __TDD__AddLongRoadSlope[-] : Demux  Outputs=[1]
  __TDD__AddRoadElev[m] : Demux  Outputs=[1]
  __TDD__LocalRoadSysSwitch[0;1] : Demux  Outputs=[1]
  __TDD__RelInflPress[Pa] : Demux  Outputs=1
  __TDD__RoadFrictionScaling[0_2] : Demux  Outputs=[1]
  AddRoadElev[m]___UNIQUE_1 : Outport  Description=|  PortDimensions=[1]  VectorParamsAs1DForOutWhenUnconnected=off
      | <name>AddRoadElev[m]</name>
      | <comment></comment>
  RoadFrictionScaling[0_2]___UNIQUE_1 : Outport  Description=|  Port=2  PortDimensions=[1]  VectorParamsAs1DForOutWhenUnconnected=off
      | <name>RoadFrictionScaling[0_2]</name>
      | <comment></comment>
  AddLongRoadSlope[-]___UNIQUE_1 : Outport  Description=|  Port=3  PortDimensions=[1]  VectorParamsAs1DForOutWhenUnconnected=off
      | <name>AddLongRoadSlope[-]</name>
      | <comment></comment>
  AddLatRoadSlope[-]___UNIQUE_1 : Outport  Description=|  Port=4  PortDimensions=[1]  VectorParamsAs1DForOutWhenUnconnected=off
      | <name>AddLatRoadSlope[-]</name>
      | <comment></comment>
  LocalRoadSysSwitch[0;1]___UNIQUE_1 : Outport  Description=|  Port=5  PortDimensions=[1]  VectorParamsAs1DForOutWhenUnconnected=off
      | <name>LocalRoadSysSwitch[0;1]</name>
      | <comment></comment>
  RelInflPress[Pa]___UNIQUE_1 : Outport  Description=|  Port=6  VectorParamsAs1DForOutWhenUnconnected=off
      | <name>RelInflPress[Pa]</name>
      | <comment></comment>
  wires:
  fromCTRL/1 -> TDBusSelector/1
  TDBusSelector/1 -> __TDD__AddRoadElev[m]/1  "<AddRoadElev[m]>"
  TDBusSelector/2 -> __TDD__RoadFrictionScaling[0_2]/1  "<RoadFrictionScaling[0_2]>"
  TDBusSelector/3 -> __TDD__AddLongRoadSlope[-]/1  "<AddLongRoadSlope[-]>"
  TDBusSelector/4 -> __TDD__AddLatRoadSlope[-]/1  "<AddLatRoadSlope[-]>"
  TDBusSelector/5 -> __TDD__LocalRoadSysSwitch[0;1]/1  "<LocalRoadSysSwitch[0;1]>"
  TDBusSelector/6 -> __TDD__RelInflPress[Pa]/1  "<RelInflPress[Pa]>"
  __TDD__AddRoadElev[m]/1 -> AddRoadElev[m]___UNIQUE_1/1  "AddRoadElev[m]"
  __TDD__RoadFrictionScaling[0_2]/1 -> RoadFrictionScaling[0_2]___UNIQUE_1/1  "RoadFrictionScaling[0_2]"
  __TDD__AddLongRoadSlope[-]/1 -> AddLongRoadSlope[-]___UNIQUE_1/1  "AddLongRoadSlope[-]"
  __TDD__AddLatRoadSlope[-]/1 -> AddLatRoadSlope[-]___UNIQUE_1/1  "AddLatRoadSlope[-]"
  __TDD__LocalRoadSysSwitch[0;1]/1 -> LocalRoadSysSwitch[0;1]___UNIQUE_1/1  "LocalRoadSysSwitch[0;1]"
  __TDD__RelInflPress[Pa]/1 -> RelInflPress[Pa]___UNIQUE_1/1  "RelInflPress[Pa]"

== system PassengerCar/Vehicle/WheelSystem/FrontRightWheelSystem/Tire/InputFromChassis ==
  fromChassis : Inport
  TDBusSelector : BusSelector  OutputSignals=VehicleBody.Pos(WorldSys)[m],VehicleBody.RotMatrix(WorldSys)[-],WheelSystem.WheelRotAxis(VehSys)[-],WheelSystem.TirePos(VehSys)[m],WheelSystem.TireVel_wrt_WorldSys(VehSys)[m/s],WheelSystem.WheelRotVel_wrt_WorldSys(VehSys)[rad/s]
  __TDD__Pos(WorldSys)[m] : Demux  Outputs=[3]
  __TDD__RotMatrix(WorldSys)[-] : Demux  Outputs=[9]
  __TDD__TirePos(VehSys)[m] : Demux  Outputs=[3]
  __TDD__TireVel_wrt_WorldSys(VehSys)[m/s] : Demux  Outputs=[3]
  __TDD__WheelRotAxis(VehSys)[-] : Demux  Outputs=[3]
  __TDD__WheelRotVel_wrt_WorldSys(VehSys)[rad/s] : Demux  Outputs=[3]
  Pos(WorldSys)[m]___UNIQUE_1 : Outport  Description=|  PortDimensions=[3]  VectorParamsAs1DForOutWhenUnconnected=off
      | <name>VehicleBody.Pos(WorldSys)[m]</name>
      | <comment></comment>
  RotMatrix(WorldSys)[-]___UNIQUE_1 : Outport  Description=|  Port=2  PortDimensions=[9]  VectorParamsAs1DForOutWhenUnconnected=off
      | <name>VehicleBody.RotMatrix(WorldSys)[-]</name>
      | <comment></comment>
  WheelRotAxis(VehSys)[-]___UNIQUE_1 : Outport  Description=|  Port=3  PortDimensions=[3]  VectorParamsAs1DForOutWhenUnconnected=off
      | <name>WheelSystem.WheelRotAxis(VehSys)[-]</name>
      | <comment></comment>
  TirePos(VehSys)[m]___UNIQUE_1 : Outport  Description=|  Port=4  PortDimensions=[3]  VectorParamsAs1DForOutWhenUnconnected=off
      | <name>WheelSystem.TirePos(VehSys)[m]</name>
      | <comment></comment>
  TireVel_wrt_WorldSys(VehSys)[m/s]___UNIQUE_1 : Outport  Description=|  Port=5  PortDimensions=[3]  VectorParamsAs1DForOutWhenUnconnected=off
      | <name>WheelSystem.TireVel_wrt_WorldSys(VehSys)[m/s]</name>
      | <comment></comment>
  WheelRotVel_wrt_WorldSys(VehSys)[rad/s]___UNIQUE_1 : Outport  Description=|  Port=6  PortDimensions=[3]  VectorParamsAs1DForOutWhenUnconnected=off
      | <name>WheelSystem.WheelRotVel_wrt_WorldSys(VehSys)[rad/s]</name>
      | <comment></comment>
  wires:
  fromChassis/1 -> TDBusSelector/1
  TDBusSelector/1 -> __TDD__Pos(WorldSys)[m]/1  "<Pos(WorldSys)[m]>"
  TDBusSelector/2 -> __TDD__RotMatrix(WorldSys)[-]/1  "<RotMatrix(WorldSys)[-]>"
  TDBusSelector/3 -> __TDD__WheelRotAxis(VehSys)[-]/1  "<WheelRotAxis(VehSys)[-]>"
  TDBusSelector/4 -> __TDD__TirePos(VehSys)[m]/1  "<TirePos(VehSys)[m]>"
  TDBusSelector/5 -> __TDD__TireVel_wrt_WorldSys(VehSys)[m/s]/1  "<TireVel_wrt_WorldSys(VehSys)[m/s]>"
  TDBusSelector/6 -> __TDD__WheelRotVel_wrt_WorldSys(VehSys)[rad/s]/1  "<WheelRotVel_wrt_WorldSys(VehSys)[rad/s]>"
  __TDD__Pos(WorldSys)[m]/1 -> Pos(WorldSys)[m]___UNIQUE_1/1  "Pos(WorldSys)[m]"
  __TDD__RotMatrix(WorldSys)[-]/1 -> RotMatrix(WorldSys)[-]___UNIQUE_1/1  "RotMatrix(WorldSys)[-]"
  __TDD__WheelRotAxis(VehSys)[-]/1 -> WheelRotAxis(VehSys)[-]___UNIQUE_1/1  "WheelRotAxis(VehSys)[-]"
  __TDD__TirePos(VehSys)[m]/1 -> TirePos(VehSys)[m]___UNIQUE_1/1  "TirePos(VehSys)[m]"
  __TDD__TireVel_wrt_WorldSys(VehSys)[m/s]/1 -> TireVel_wrt_WorldSys(VehSys)[m/s]___UNIQUE_1/1  "TireVel_wrt_WorldSys(VehSys)[m/s]"
  __TDD__WheelRotVel_wrt_WorldSys(VehSys)[rad/s]/1 -> WheelRotVel_wrt_WorldSys(VehSys)[rad/s]___UNIQUE_1/1  "WheelRotVel_wrt_WorldSys(VehSys)[rad/s]"

== system PassengerCar/Vehicle/WheelSystem/FrontRightWheelSystem/Tire/InputFromWheel ==
  fromWheel : Inport
  TDBusSelector : BusSelector  OutputSignals=RotSpd[rad/s]
  __TDD__RotSpd[rad/s] : Demux  Outputs=[1]
  RotSpd[rad/s]___UNIQUE_1 : Outport  Description=|  PortDimensions=[1]  VectorParamsAs1DForOutWhenUnconnected=off
      | <name>RotSpd[rad/s]</name>
      | <comment></comment>
  wires:
  fromWheel/1 -> TDBusSelector/1
  TDBusSelector/1 -> __TDD__RotSpd[rad/s]/1  "<RotSpd[rad/s]>"
  __TDD__RotSpd[rad/s]/1 -> RotSpd[rad/s]___UNIQUE_1/1  "RotSpd[rad/s]"
